simulink model "TrayectoriaEvitarObstaculos"  (R2023b)
settings: Solver=FixedStepAuto  StartTime=0.0  StopTime=200  RelTol=1e-3  EnableMultiTasking=on
model workspace (MAT data in the model file):
  d = 0.18
libraries: slpidlib x1
settings Model: ExtModeTrigDuration=2  Creator=Enrique  LastModifiedBy=Enrique
settings OptimizationCC: EnhancedBackFolding=on  PassReuseOutputArgsAs=Individual arguments  ZeroExternalMemoryAtStartup=off  ZeroInternalMemoryAtStartup=off  MaxStackSize=64  OptimizeBlockOrder=speed  DifferentSizesBufferReuse=on  EfficientTunableParamExpr=on
settings DebuggingCC: AlgebraicLoopMsg=none  ParameterTunabilityLossMsg=error
settings HardwareCC: ProdBitPerInt=16  ProdBitPerPointer=16  ProdBitPerSizeT=16  ProdBitPerPtrDiffT=16  ProdLargestAtomicFloat=None  ProdWordSize=8  ProdHWDeviceType=Atmel->AVR  UseEmbeddedCoderFeatures=off  UseSimulinkCoderFeatures=off
settings SFSimCC: MATLABDynamicMemAlloc=off
settings RTWCC: Description=Embedded Coder  SystemTargetFile=ert.tlc  HardwareBoard=Arduino Mega 2560  TemplateMakefile=ert_default_tmf  Toolchain=Arduino AVR  BuildConfiguration=Faster Runs
settings CodeAppCC: ForceParamTrailComments=on  IgnoreCustomStorageClasses=off  OperatorAnnotations=on  SimulinkDataObjDesc=on  SFDataObjDesc=on  MangleLength=10  InsertBlockDesc=on
settings ERTTargetCC: SupportContinuousTime=on  SupportNonInlinedSFcns=on  SupportVariableSizeSignals=on  ExtModeTransport=3  ExtModeStaticAlloc=on  ExtModeAutomaticAllocSize=off  ExtModeStaticAllocSize=2048  ExtModeMexFile=ext_xcp  ExtModeIntrfLevel=Level2 - Open

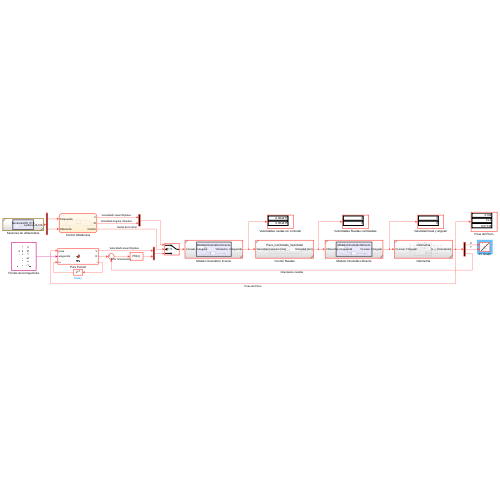
[thumbnail: Simulink's stored preview of the top-level diagram]
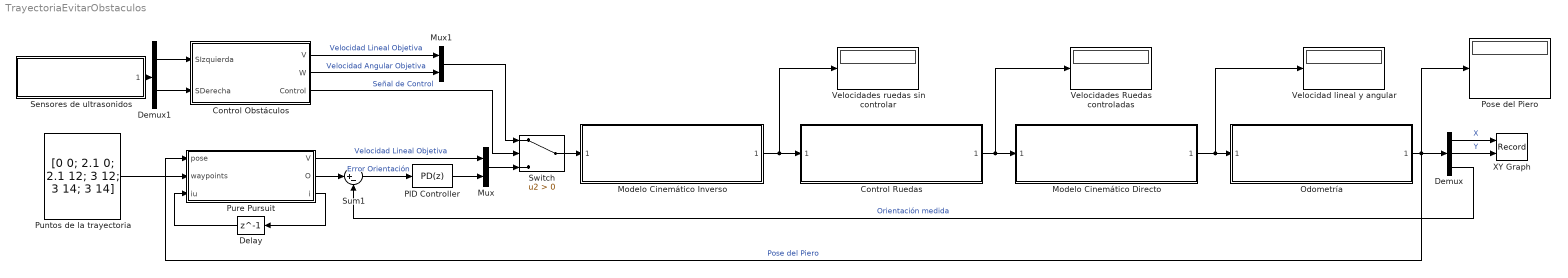
== system TrayectoriaEvitarObstaculos ==
  Control Obstáculos : Stateflow chart  TreatAsAtomicUnit=on
  Control Ruedas : Subsystem  ReferencedSubsystem=Piero_Controlado_Velocidad
  Delay : Delay  DelayLength=1
  Demux : Demux  Outputs=3
  Demux1 : Demux  Outputs=2
  Modelo Cinemático Directo : Subsystem  ReferencedSubsystem=ModeloCinematicoDirecto
  Modelo Cinemático Inverso : Subsystem  ReferencedSubsystem=ModeloCinematicoInverso
  Mux : Mux  Inputs=2
  Mux1 : Mux  Inputs=2
  Odometría : Subsystem  ReferencedSubsystem=Odometria
  PID Controller : slpidlib/PID Controller  Controller=PD  Form=Parallel  TimeDomain=Discrete-time  UseExternalTs=off  SampleTime=0.01  IntegratorMethod=Forward Euler  FilterMethod=Forward Euler  ControllerParametersSource=internal  P=2.86029939965115  I=0.546838423026858  UseKiTs=off  D=0.802889874286159  N=15.3561441293328  UseFilter=on  TunerSelectOption=Transfer Function Based (PID Tuner App)  InitialConditionSource=internal  InitialConditionForIntegrator=0  InitialConditionForFilter=0  DifferentiatorICPrevScaledInput=0  ExternalReset=none  TrackingMode=off  Kt=1  LimitOutput=off  SatLimitsSource=internal  UpperSaturationLimit=inf  LowerSaturationLimit=-inf  LinearizeAsGain=on  AntiWindupMode=none  Kb=1  LimitIntegrator=off  UpperIntegratorSaturationLimit=inf  LowerIntegratorSaturationLimit=-inf  POutMin=[]  POutMax=[]  IOutMin=[]  IOutMax=[]  DOutMin=[]  DOutMax=[]  NOutMin=[]  NOutMax=[]  SumOutMin=[]  SumOutMax=[]  SaturationOutMin=[]  SaturationOutMax=[]  PParamMin=[]  PParamMax=[]  IParamMin=[]  IParamMax=[]  DParamMin=[]  DParamMax=[]  NParamMin=[]  NParamMax=[]  KbParamMin=[]  KbParamMax=[]  KtParamMin=[]  KtParamMax=[]  KbOutMin=[]  KbOutMax=[]  KtOutMin=[]  KtOutMax=[]  IntegratorOutMin=[]  IntegratorOutMax=[]  FilterOutMin=[]  FilterOutMax=[]  SumI1OutMin=[]  SumI1OutMax=[]  SumI2OutMin=[]  SumI2OutMax=[]  SumI3OutMin=[]  SumI3OutMax=[]  SumI4OutMin=[]  SumI4OutMax=[]  SumDOutMin=[]  SumDOutMax=[]  DifferentiatorOutMin=[]  DifferentiatorOutMax=[]  FilterDiffOutCoefMin=[]  FilterDiffOutCoefMax=[]  ReciprocalOutMin=[]  ReciprocalOutMax=[]  SumDenOutMin=[]  SumDenOutMax=[]  SumNumOutMin=[]  SumNumOutMax=[]  DivideOutMin=[]  DivideOutMax=[]  UdiffTsProdOutMin=[]  UdiffTsProdOutMax=[]  NTsProdOutMin=[]  NTsProdOutMax=[]  UintegralTsProdOutMin=[]  UintegralTsProdOutMax=[]  UngainTsProdOutMin=[]  UngainTsProdOutMax=[]  ClampingZeroOutDataTypeStr=Inherit: Inherit via back propagation  ClampingZeroOutMin=[]  ClampingZeroOutMax=[]  FilterDenConstantOutDataTypeStr=Inherit: Inherit via back propagation  FilterDenConstantOutMin=[]  FilterDenConstantOutMax=[]  PCopyOutDataTypeStr=Inherit: Inherit via back propagation  PCopyOutMin=[]  PCopyOutMax=[]  NCopyOutDataTypeStr=Inherit: Inherit via back propagation  NCopyOutMin=[]  NCopyOutMax=[]  IntegratorContinuousStateAttributes=''  IntegratorStateMustResolveToSignalObject=off  IntegratorRTWStateStorageClass=Auto  FilterContinuousStateAttributes=''  FilterStateMustResolveToSignalObject=off  FilterRTWStateStorageClass=Auto  ParallelPVariant=InternalParameters  IdealPVariant=Disabled  IVariant=Disabled  DVariant=InternalParameters  IntegratorVariant=Disabled  SatVariant=Disabled  AWVariant=Disabled  PCopyVariant=Disabled  TRVariant=Disabled  FdbkBlocksVariant=Forward  IdealPFdbkVariant=Disabled  SatFdbkVariant=Disabled  DerivativeFilterVariant=ForwardEulerFilter  NVariant=InternalParameters  NCopyVariant=Disabled  FilterICVariant=InternalICsFilter  IntegratorICVariant=Disabled  ExternalResetVariant=Disabled  TRSumVariant=Passthrough  SumFdbkVariant=Disabled  SumVariant=Sum_PD  TsampFilterVariant=InternalTs  TsampNgainVariant=Passthrough  TsampIntegralVariant=Disabled_SignalSpec  ExternalSaturationOutDataTypeStr=Inherit: Same as second input
  Pose del Piero : Display
  Puntos de la trayectoria : Constant  Value=[0 0; 2.1 0; 2.1 12; 3 12; 3 14; 3 14]
  Pure Pursuit : MATLAB Function  TreatAsAtomicUnit=on
  Sensores de ultrasonidos : Subsystem  ReferencedSubsystem=SensoresUS_016
  Sum1 : Sum  Inputs=|+-
  Switch : Switch  Criteria=u2 > Threshold  SaturateOnIntegerOverflow=off  InputSameDT=off
  Velocidad lineal y angular : Display
  Velocidades Ruedas controladas : Display
  Velocidades ruedas sin controlar : Display
  XY Graph : Record  FileSettingsInternal="{\"entries\":[{\"content\":{\"excelSettings\":{\"content\":{},\"type\":\"Streamout.ExcelSettings\"}},\"type\":\"Streamout.FileSettingStorage\",\"uuid\":\"\"}],\"packageUris\":[\"http:\\/\\/schema.mathworks.com\\/mf0\\/streamout_blocks\\/R2020a\"],\"version\":\"1.0\"}"  Layout=[1 1]  SignalsInternal="{\"entries\":[{\"content\":{\"signals\":[{\"content\":{\"blockPath\":[],\"dimensions\":[1],\"domain\":\"\",\"lineColor\":\"#a2142f\",\"plots\":[ 1 ],\"port\":1,\"sid\":[\"53\"],\"signalID\":1,\"signalName\":\"X\"},\"type\":\"RecordBlkView.Signal\",\"uuid\":\"\"},{\"content\":{\"blockPath\":[],\"dimensions\":[1],\"domain\":\"\",\"lineColor\":\"#139fff\",\"plots\":[ 1 ],\"port\":2,\"sid\":[\"53\"],\"signalID\":2,\"signalName\":\"Y\"},\"type\":\"RecordBlkView.Signal\",\"uuid\":\"\"}]},\"type\":\"RecordBlkView.InputSignals\",\"uuid\":\"\"}],\"packageUris\":[\"http:\\/\\/schema.mathworks.com\\/mf0\\/streamout_blocks\\/R2020a\"],\"version\":\"1.0\"}"  VisualizationBindings="{\"xyplotplugin\":{\"info\":[{\"series\":[{\"bindingParametersList\":[{\"parameter\":\"X-Axis\",\"signalID\":1,\"signalName\":\"X\"},{\"parameter\":\"Y-Axis\",\"signalID\":2,\"signalName\":\"Y\"}],\"seriesID\":0}],\"subplotID\":1}]}}"  CompatibilityTag=XY
  wires:
  Modelo Cinemático Inverso/1 -> Velocidades ruedas sin controlar/1, Control Ruedas/1
  Control Ruedas/1 -> Modelo Cinemático Directo/1, Velocidades Ruedas controladas/1
  Modelo Cinemático Directo/1 -> Odometría/1, Velocidad lineal y angular/1
  Odometría/1 -> Pure Pursuit/1(pose), Pose del Piero/1, Demux/1  "Pose del Piero"
  Demux/1 -> XY Graph/1  "X"
  Pure Pursuit/1(V) -> Mux/1  "Velocidad Lineal Objetiva"
  Demux/2 -> XY Graph/2  "Y"
  Puntos de la trayectoria/1 -> Pure Pursuit/2(waypoints)
  Control Obstáculos/1(V) -> Mux1/1  "Velocidad Lineal Objetiva"
  Control Obstáculos/2(W) -> Mux1/2  "Velocidad Angular Objetiva"
  Control Obstáculos/3(Control) -> Switch/2  "Señal de Control"
  Sensores de ultrasonidos/1 -> Demux1/1
  Demux1/1 -> Control Obstáculos/1(SIzquierda)
  Demux1/2 -> Control Obstáculos/2(SDerecha)
  Pure Pursuit/3(i) -> Delay/1
  Delay/1 -> Pure Pursuit/3(iu)
  Sum1/1 -> PID Controller/1  "Error Orientación"
  Pure Pursuit/2(O) -> Sum1/1
  PID Controller/1 -> Mux/2
  Demux/3 -> Sum1/2  "Orientación medida"
  Switch/1 -> Modelo Cinemático Inverso/1
  Mux/1 -> Switch/3
  Mux1/1 -> Switch/1

== stateflow chart TrayectoriaEvitarObstaculos/Control Obstáculos ==
  state SinObstaculos
    V = 0;
    W = 0;
    Control = 0;
  state ObstaculoIzquierda
    V = 0.1;
    W = -pi/2;
    Control = 1;
  state ObstaculoDerecha
    V = 0.1;
    W = pi/2;
    Control = 1;
  (default) -> SinObstaculos
  SinObstaculos -> ObstaculoIzquierda [order 1] : [SIzquierda < 40]
  SinObstaculos -> ObstaculoDerecha [order 2] : [SDerecha < 40]
  ObstaculoIzquierda -> SinObstaculos : [SIzquierda > 50]
  ObstaculoDerecha -> SinObstaculos : [SDerecha > 50]
  data: V output; W output; Control output; SIzquierda input; SDerecha input

== matlab function TrayectoriaEvitarObstaculos/Pure Pursuit ==
  data: pose input; V output; waypoints input; O output; i output; iu input
function [V,O, i] = fcn(pose, waypoints, iu)

% Margen de distancia
LA = 0.1;

%Inicializamos variables
V = 0.2;
O = 0;
i = 0;

if(isempty(iu) || iu < 1)
    iu = 1;
end

% Extraemos la posición
x = pose(1);
y = pose(2);
o = pose(3);

if(length(waypoints) >= iu)
    distancia = sqrt((waypoints(iu,1)-x)^2 + (waypoints(iu,2)-y)^2);

    if(distancia > LA)
        O = atan2(waypoints(iu,2)-y, waypoints(iu,1)-x);
        V = 0.2;
    else
        iu = iu+1;
    end    
else
    O = 0;
    V = 0;
end

i = iu;
